simulink model "joystick_test"  (R2023a)
settings: Solver=ode2  StartTime=0.0  StopTime=inf  FixedStep=0.002  RelTol=1e-3  EnableMultiTasking=on
libraries: quarc_library x3, simulink x2
settings Model: SimulationMode=external  ExtModeTrigDuration=10000  Creator=mbohra  LastModifiedBy=Admin
settings SolverCC: AlgebraicLoopSolver=TrustRegion  PositivePriorityOrder=on
settings DataIOCC: SaveOutput=off  SignalLogging=off  DSMLogging=off  SaveTime=off  ReturnWorkspaceOutputs=off
settings DebuggingCC: UnconnectedInputMsg=warning  UnconnectedOutputMsg=warning  UnconnectedLineMsg=warning  ArithmeticOperatorsInVariantConditions=warning
settings ModelReferenceCC: EnableRefExpFcnMdlSchedulingChecks=on
settings SFSimCC: CustomCodeUndefinedFunction=UseInterfaceOnly
settings RTWCC: Description=QUARC Win64 Target Using Toolchain  SystemTargetFile=quarc_win64.tlc  TemplateMakefile=quarc_default_tmf  Toolchain=QUARC win64 | nmake (64-bit Windows)  BuildConfiguration=Faster Runs
settings STFCustomTargetCC: SystemTargetFile=quarc_win64.tlc
settings GRTTargetCC: ParMdlRefBuildCompliant=off  CompOptLevelCompliant=off  CombineOutputUpdateFcns=off  MatFileLogging=off  CPPClassGenCompliant=off  GRTInterface=on  ExtMode=on  ExtModeMexFile=quarc_comm

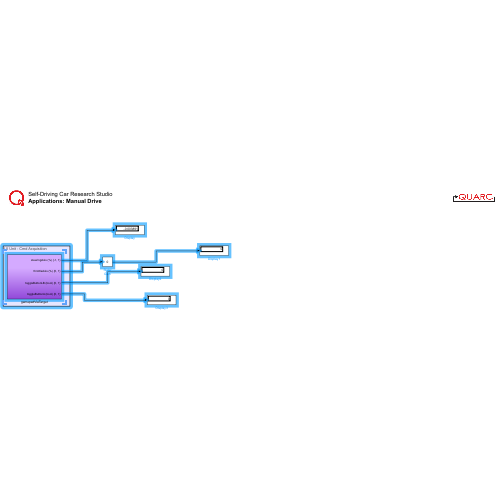
[thumbnail: Simulink's stored preview of the top-level diagram]
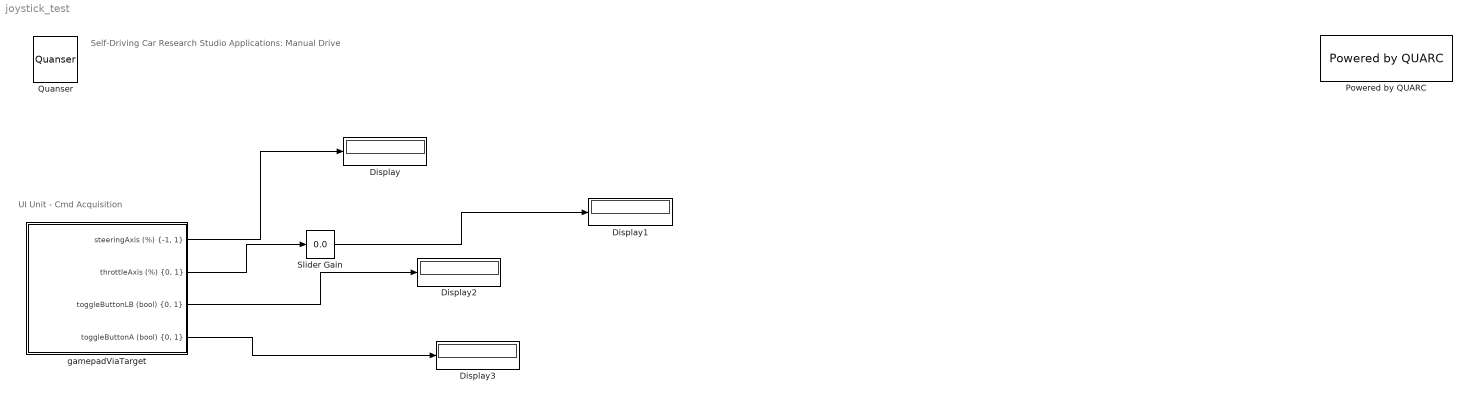
== system joystick_test ==
  note: UI Unit - Cmd Acquisition
  note: Self-Driving Car Research Studio
      | Applications: Manual Drive
  Display{,1..3} (4 alike) : Display
  Powered by QUARC : quarc_library/Logos/Powered by QUARC
  Quanser : quarc_library/Logos/Quanser
  Slider Gain : simulink/Math Operations/Slider Gain  gain=0.0  low=-0.5  high=0.5
  gamepadViaTarget : Subsystem
  wires:
  gamepadViaTarget/1("steeringAxis (%) {-1, 1}") -> Display/1
  gamepadViaTarget/3("toggleButtonLB (bool) {0, 1}") -> Display2/1
  gamepadViaTarget/4("toggleButtonA (bool) {0, 1}") -> Display3/1
  gamepadViaTarget/2("throttleAxis (%) {0, 1}") -> Slider Gain/1
  Slider Gain/1 -> Display1/1

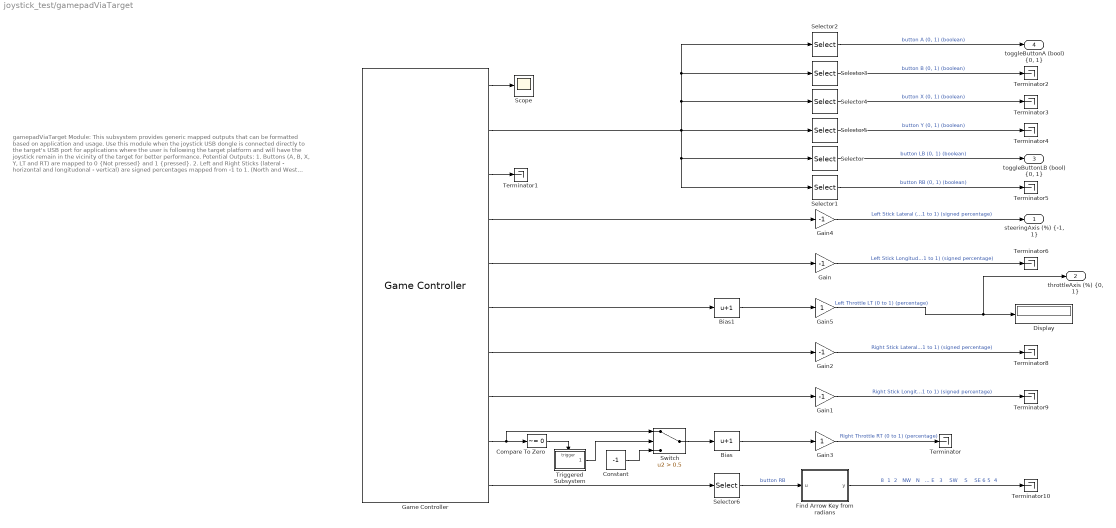
== system joystick_test/gamepadViaTarget ==
  note: gamepadViaTarget Module:
      |
      | This subsystem provides generic mapped outputs that can be formatted based on application and usage. Use this module when the joystick USB dongle is connected directly to the target's USB port for applications where the user is following the target platform and will have the joystick remain in the vicinity of the target for better performance.
      |
      | Potential Outputs:
      |
      | 1. Buttons (A, B, X, Y, LT and RT) are mapped to 0 {Not pressed} and 1 {pressed}.
      |
      | 2. Left and Right Sticks (lateral - horizontal and longitudonal - vertical) are signed percentages mapped from -1 to 1. (North and West directions are positive)
      |
      | 3. Throttle (RT and LT) are mapped from 0 to 1.
      |
      | 4. Arrow keys are mapped to constants 1 to 8 starting from North and incrementing clockwise up to North West. A value of 0 implies no keys are pressed.
      |
      | 5. The NEW signal triggers a high (1) pulse whenever a value on any of the gamepad's keys changes.
      |
      | NOTE: The Gamepad F710 dongle MUST be plugged into the target's USB port to use this module.
  Bias : Bias  Bias=1  SaturateOnIntegerOverflow=off
  Bias1 : Bias  Bias=1  SaturateOnIntegerOverflow=off
  Compare To Zero : simulink/Logic and Bit Operations/Compare To Zero  relop=~=  OutDataTypeStr=boolean
  Constant : Constant  Value=-1
  Display : Display
  Find Arrow Key from radians : MATLAB Function  TreatAsAtomicUnit=on
  Gain{,1..2,4} (4 alike) : Gain  Gain=-1
  Gain3 : Gain
  Gain5 : Gain
  Game Controller : quarc_library/Devices/Peripherals/Target/Game Controller  controller=2  buffer_size=12  deadzone=[]  saturation=[]  sample_time=qc_get_step_size  auto_center=off  enabled=on
      settings: SourceProductName=QUARC Targets
  Scope : Scope
  Selector : Selector  InputPortWidth=32  IndexOptions=Index vector (dialog)  Indices=[5]  OutputSizes=1
  Selector1 : Selector  InputPortWidth=32  IndexOptions=Index vector (dialog)  Indices=[6]  OutputSizes=1
  Selector2 : Selector  InputPortWidth=32  IndexOptions=Index vector (dialog)  Indices=[1]  OutputSizes=1
  Selector3 : Selector  InputPortWidth=32  IndexOptions=Index vector (dialog)  Indices=[2]  OutputSizes=1
  Selector4 : Selector  InputPortWidth=32  IndexOptions=Index vector (dialog)  Indices=[3]  OutputSizes=1
  Selector5 : Selector  InputPortWidth=32  IndexOptions=Index vector (dialog)  Indices=[4]  OutputSizes=1
  Selector6 : Selector  InputPortWidth=4  IndexOptions=Index vector (dialog)  Indices=[1]  OutputSizes=1
  Switch : Switch  Criteria=u2 > Threshold  Threshold=0.5  SaturateOnIntegerOverflow=off  InputSameDT=off
  Terminator{,1..6,8..10} (10 alike) : Terminator
  Triggered Subsystem : Subsystem  TreatAsAtomicUnit=on
  "steeringAxis (%) {-1, 1}" : Outport  VectorParamsAs1DForOutWhenUnconnected=off
  "throttleAxis (%) {0, 1}" : Outport  Port=2  VectorParamsAs1DForOutWhenUnconnected=off
  "toggleButtonLB (bool) {0, 1}" : Outport  Port=3  VectorParamsAs1DForOutWhenUnconnected=off
  "toggleButtonA (bool) {0, 1}" : Outport  Port=4  VectorParamsAs1DForOutWhenUnconnected=off
  wires:
  Bias1/1 -> Gain5/1
  Game Controller/6 -> Bias1/1
  Game Controller/10 -> Selector6/1
  Selector5/1 -> Terminator4/1  "button Y (0, 1) (boolean)"
  Selector4/1 -> Terminator3/1  "button X (0, 1) (boolean)"
  Selector3/1 -> Terminator2/1  "button B (0, 1) (boolean)"
  Game Controller/1 -> Scope/1
  Game Controller/5 -> Gain/1
  Game Controller/4 -> Gain4/1
  Game Controller/8 -> Gain1/1
  Game Controller/7 -> Gain2/1
  Game Controller/2 -> Selector1/1, Selector/1, Selector5/1, Selector2/1, Selector3/1, Selector4/1
  Bias/1 -> Gain3/1
  Gain2/1 -> Terminator8/1  "Right Stick Lateral (-1 to 1) (signed percentage)"
  Gain1/1 -> Terminator9/1  "Right Stick Longitudonal (-1 to 1) (signed percentage)"
  Gain/1 -> Terminator6/1  "Left Stick Longitudonal (-1 to 1) (signed percentage)"
  Selector1/1 -> Terminator5/1  "button RB (0, 1) (boolean)"
  Selector/1 -> "toggleButtonLB (bool) {0, 1}"/1  "button LB (0, 1) (boolean)"
  Selector2/1 -> "toggleButtonA (bool) {0, 1}"/1  "button A (0, 1) (boolean)"
  Gain4/1 -> "steeringAxis (%) {-1, 1}"/1  "Left Stick Lateral (-1 to 1) (signed percentage)"
  Selector6/1 -> Find Arrow Key from radians/1(u)  "button RB"
  Find Arrow Key from radians/1(y) -> Terminator10/1  "8 \t\t\t1\t\t\t 2   NW\t  N\t\t  NE \t\t 7     W\t\t0\t\t  E   3     SW\t   S\t\t   SE 6\t\t\t5\t\t\t 4"
  Game Controller/3 -> Terminator1/1
  Switch/1 -> Bias/1
  Game Controller/9 -> Switch/1, Compare To Zero/1
  Triggered Subsystem/1(Enabled) -> Switch/2
  Constant/1 -> Switch/3
  Compare To Zero/1 -> Triggered Subsystem/Trigger
  Gain5/1 -> "throttleAxis (%) {0, 1}"/1, Display/1  "Left Throttle LT (0 to 1) (percentage)"
  Gain3/1 -> Terminator/1  "Right Throttle RT (0 to 1) (percentage)"

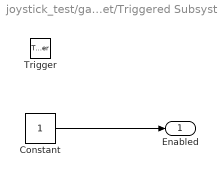
== system joystick_test/gamepadViaTarget/Triggered Subsystem ==
  Trigger : TriggerPort  VariantControl=Variant
  Constant : Constant
  Enabled : Outport  InitialOutput=[0]
  wires:
  Constant/1 -> Enabled/1

== matlab function joystick_test/gamepadViaTarget/Find Arrow Key from radians ==
  data: u input; y output
function y = fcn(u)

% the input signal gives the positon of the arrow keys pressed on the gamepad
% in radians circulating clockwise. Thus, up arrow alone is 0, right would be
% pi/2, and both up and right arrows pressed simultaneously is pi/4.
% 
% Given the input signal, convert to degrees for ease, then subtract the 
% vector 45*[0 1 2 3 4 5 6 7] to find smallest error corresponding to arrow
% pressed. 
if u == -1
    y = 0;
else
    [~, y] = min(abs((u*360/(2*pi)) - 45*[0 1 2 3 4 5 6 7]));
end
